simulink model "sim_statefeedback"  (R2023b)
settings: Solver=VariableStepAuto  StartTime=0.0  StopTime=TSim  RelTol=1e-3
undefined symbols (not defined in the file): dampingCoeff, freqDist, initPos, initVel, K, magDist, mass, phaseDist, springCoeff
libraries: simulink x2
settings Model: Creator=uos  LastModifiedBy=hblee

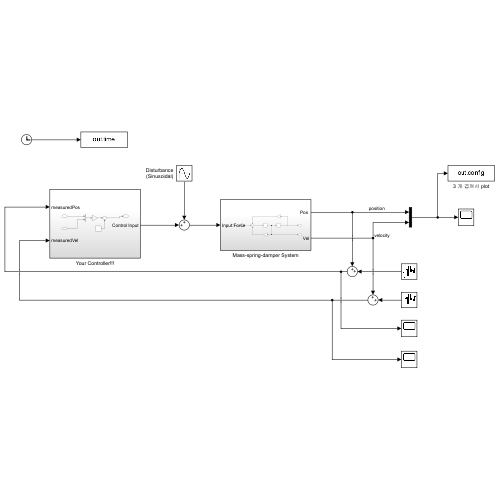
[thumbnail: Simulink's stored preview of the top-level diagram]
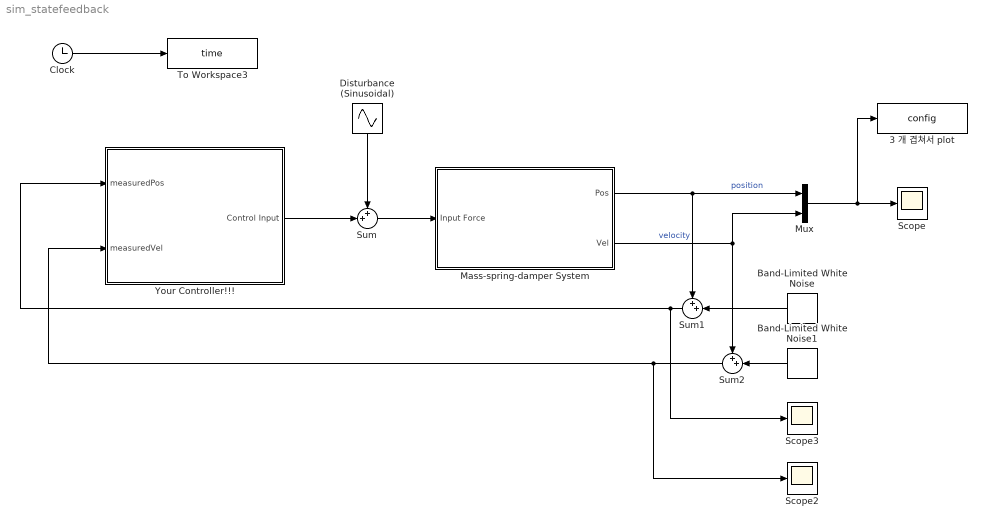
== system sim_statefeedback ==
  3 개 겹쳐서 plot : ToWorkspace  VariableName=config  SampleTime=-1
  Band-Limited White Noise : simulink/Sources/Band-Limited White Noise  Cov=powerNoise  Ts=0.001  seed=[23341]
  Band-Limited White Noise1 : simulink/Sources/Band-Limited White Noise  Cov=powerNoise  Ts=0.001  seed=[23341]
  Clock : Clock
  Disturbance (Sinusoidal) : Sin  Amplitude=magDist  Bias=phaseDist  Frequency=freqDist  SampleTime=0
  Mass-spring-damper System : Subsystem
  Mux : Mux  Inputs=2
  Scope : Scope
  Scope2 : Scope
  Scope3 : Scope
  Sum : Sum  Inputs=++|
  Sum1 : Sum  Inputs=++|
  Sum2 : Sum  Inputs=++|
  To Workspace3 : ToWorkspace  VariableName=time  SampleTime=-1
  Your Controller!!! : Subsystem
  wires:
  Mass-spring-damper System/2(Vel) -> Mux/2, Sum2/1  "velocity"
  Sum/1 -> Mass-spring-damper System/1("Input Force ")
  Your Controller!!!/1(Control Input) -> Sum/2
  Sum1/1 -> Scope3/1, Your Controller!!!/1(measuredPos)
  Sum2/1 -> Scope2/1, Your Controller!!!/2(measuredVel)
  Band-Limited White Noise/1 -> Sum1/2
  Band-Limited White Noise1/1 -> Sum2/2
  Disturbance (Sinusoidal)/1 -> Sum/1
  Clock/1 -> To Workspace3/1
  Mass-spring-damper System/1("Pos ") -> Sum1/1, Mux/1  "position"
  Mux/1 -> 3 개 겹쳐서 plot/1, Scope/1

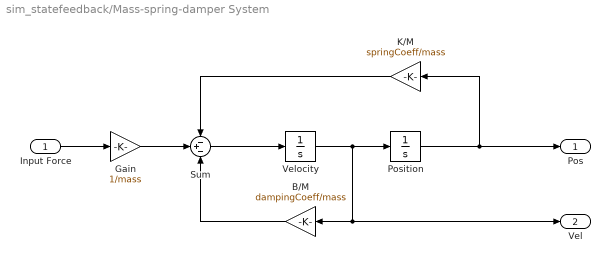
== system sim_statefeedback/Mass-spring-damper System ==
  "Input Force " : Inport
  B/M : Gain  Gain=dampingCoeff/mass
  Gain : Gain  Gain=1/mass
  K/M : Gain  Gain=springCoeff/mass
  Position : Integrator  InitialCondition=initPos
  Sum : Sum  Inputs=-+-
  Velocity : Integrator  InitialCondition=initVel
  "Pos " : Outport
  Vel : Outport  Port=2
  wires:
  Velocity/1 -> Vel/1, B/M/1, Position/1
  Gain/1 -> Sum/2
  "Input Force "/1 -> Gain/1
  Position/1 -> "Pos "/1, K/M/1
  K/M/1 -> Sum/1
  B/M/1 -> Sum/3
  Sum/1 -> Velocity/1

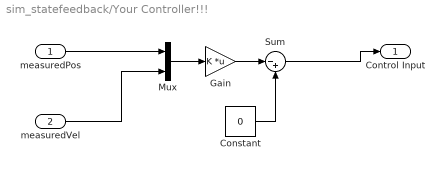
== system sim_statefeedback/Your Controller!!! ==
  measuredPos : Inport
  measuredVel : Inport  Port=2
  Constant : Constant  Value=0
  Gain : Gain  Gain=K  Multiplication=Matrix(K*u)
  Mux : Mux  Inputs=2
  Sum : Sum  Inputs=|-+
  Control Input : Outport
  wires:
  Mux/1 -> Gain/1
  Gain/1 -> Sum/1
  Sum/1 -> Control Input/1
  Constant/1 -> Sum/2
  measuredPos/1 -> Mux/1
  measuredVel/1 -> Mux/2
